simulink subsystem "system_outputs"  (R2022b)
settings: Solver=VariableStepAuto  StartTime=0.0  StopTime=10.0  RelTol=1e-3
libraries: mbedblockslib x1
settings Model: Creator=micha  LastModifiedBy=micha
settings ModelReferenceCC: EnableRefExpFcnMdlSchedulingChecks=on

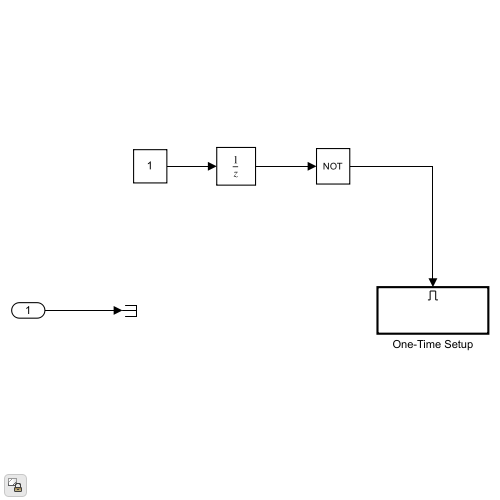
[thumbnail: Simulink's stored preview of the top-level diagram]
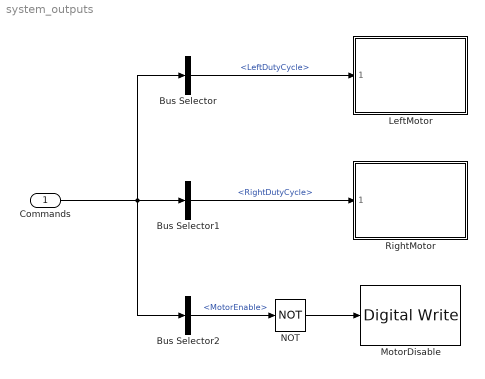
== system system_outputs ==
  Commands : Inport
  Bus Selector : BusSelector  OutputSignals=LeftDutyCycle
  Bus Selector1 : BusSelector  OutputSignals=RightDutyCycle
  Bus Selector2 : BusSelector  OutputSignals=MotorEnable
  LeftMotor : Subsystem  ReferencedSubsystem=motor_drive  pwm_pin=D10  dir_pin=D3  flip_direction=off
  MotorDisable : mbedblockslib/Digital Write  Pin=D8  Direction=output
      settings: LibrarySourceBlock=stmnucleorootlib/Common/Digital Write
  NOT : Logic  Operator=NOT  AllPortsSameDT=off  OutDataTypeStr=boolean
  RightMotor : Subsystem  ReferencedSubsystem=motor_drive  pwm_pin=D5  dir_pin=D4  flip_direction=on
  wires:
  Commands/1 -> Bus Selector1/1, Bus Selector2/1, Bus Selector/1
  NOT/1 -> MotorDisable/1
  Bus Selector2/1 -> NOT/1  "<MotorEnable>"
  Bus Selector1/1 -> RightMotor/1  "<RightDutyCycle>"
  Bus Selector/1 -> LeftMotor/1  "<LeftDutyCycle>"
